simulink model "Lin_cartmodel"  (R2019b)
settings: Solver=VariableStepAuto  StartTime=0.0  StopTime=10.0  RelTol=1e-3
values from neighbouring files (symbols this model uses):
  A = Ab    [mainfile_solution.m]
  B = Bb    [mainfile_solution.m]
  C = Cb    [mainfile_solution.m]
  controller_enabled = 1    [mainfile_solution.m]
  K = place(A,B,p)    [mainfile_solution.m]
  L = place(A',C',p)'    [mainfile_solution.m]
  use_state_estimates = 1    [mainfile_solution.m]
  x0 = x0b    [mainfile_solution.m]
  x_bar = xb_bar    [mainfile_solution.m]
settings Model: Creator=n9182250  LastModifiedBy=n9182250
settings DebuggingCC: ArithmeticOperatorsInVariantConditions=warning
settings SFSimCC: CustomCodeUndefinedFunction=UseInterfaceOnly

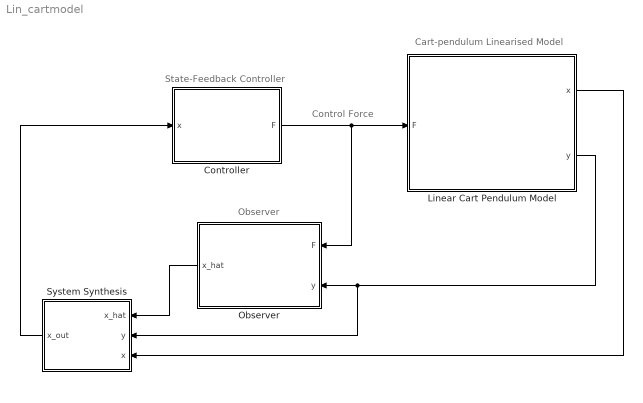
== system Lin_cartmodel ==
  note: Cart-pendulum Linearised Model
  note: Control Force
  note: State-Feedback Controller
  note: Observer
  Controller : Subsystem
  Linear Cart Pendulum Model : Subsystem
  Observer : Subsystem
  System Synthesis : Subsystem
  wires:
  Controller/1(F) -> Observer/1(F), Linear Cart Pendulum Model/1(F)
  Linear Cart Pendulum Model/2(y) -> System Synthesis/2(y), Observer/2(y)
  Observer/1(x_hat) -> System Synthesis/1(x_hat)
  Linear Cart Pendulum Model/1("x ") -> System Synthesis/3(x)
  System Synthesis/1(x_out) -> Controller/1(x)

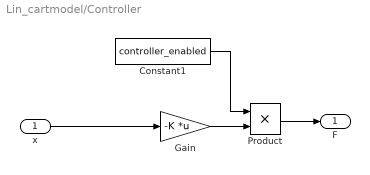
== system Lin_cartmodel/Controller ==
  x : Inport
  Constant1 : Constant  Value=controller_enabled
  Gain : Gain  Gain=-K  Multiplication=Matrix(K*u)
  Product : Product
  F : Outport
  wires:
  x/1 -> Gain/1
  Constant1/1 -> Product/1
  Gain/1 -> Product/2
  Product/1 -> F/1

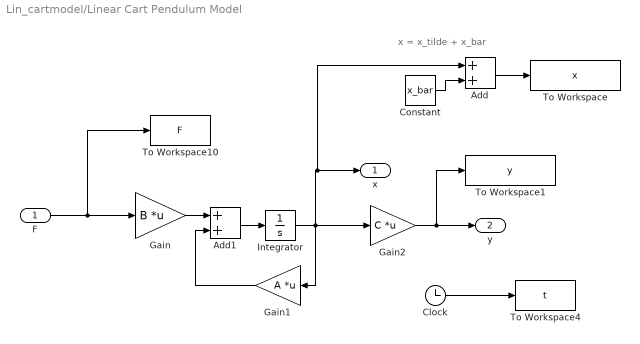
== system Lin_cartmodel/Linear Cart Pendulum Model ==
  note: x = x_tilde + x_bar
  F : Inport
  Add : Sum
  Add1 : Sum
  Clock : Clock
  Constant : Constant  Value=x_bar
  Gain : Gain  Gain=B  Multiplication=Matrix(K*u)
  Gain1 : Gain  Gain=A  Multiplication=Matrix(K*u)
  Gain2 : Gain  Gain=C  Multiplication=Matrix(K*u)
  Integrator : Integrator  InitialCondition=x0-x_bar
  To Workspace : ToWorkspace  VariableName=x  SampleTime=-1
  To Workspace1 : ToWorkspace  VariableName=y  SampleTime=-1
  To Workspace10 : ToWorkspace  VariableName=F  SampleTime=-1
  To Workspace4 : ToWorkspace  VariableName=t  SampleTime=-1
  "x " : Outport  VectorParamsAs1DForOutWhenUnconnected=off
  y : Outport  Port=2  VectorParamsAs1DForOutWhenUnconnected=off
  wires:
  F/1 -> To Workspace10/1, Gain/1
  Clock/1 -> To Workspace4/1
  Add/1 -> To Workspace/1
  Gain/1 -> Add1/1
  Gain1/1 -> Add1/2
  Add1/1 -> Integrator/1
  Integrator/1 -> Add/1, "x "/1, Gain2/1, Gain1/1
  Gain2/1 -> To Workspace1/1, y/1
  Constant/1 -> Add/2

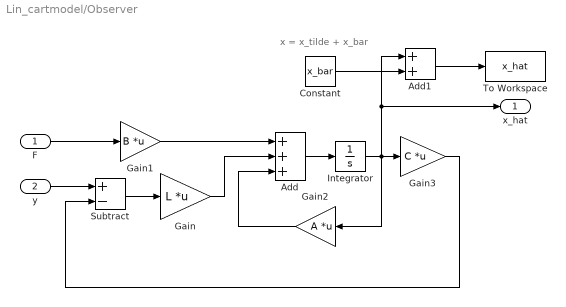
== system Lin_cartmodel/Observer ==
  note: x = x_tilde + x_bar
  F : Inport
  y : Inport  Port=2
  Add : Sum  Inputs=+++
  Add1 : Sum
  Constant : Constant  Value=x_bar
  Gain : Gain  Gain=L  Multiplication=Matrix(K*u)
  Gain1 : Gain  Gain=B  Multiplication=Matrix(K*u)
  Gain2 : Gain  Gain=A  Multiplication=Matrix(K*u)
  Gain3 : Gain  Gain=C  Multiplication=Matrix(K*u)
  Integrator : Integrator
  Subtract : Sum  Inputs=+-
  To Workspace : ToWorkspace  VariableName=x_hat  SampleTime=-1
  x_hat : Outport  VectorParamsAs1DForOutWhenUnconnected=off
  wires:
  y/1 -> Subtract/1
  Subtract/1 -> Gain/1
  F/1 -> Gain1/1
  Gain1/1 -> Add/1
  Gain/1 -> Add/2
  Add/1 -> Integrator/1
  Gain2/1 -> Add/3
  Gain3/1 -> Subtract/2
  Constant/1 -> Add1/2
  Integrator/1 -> Add1/1, x_hat/1, Gain2/1, Gain3/1
  Add1/1 -> To Workspace/1

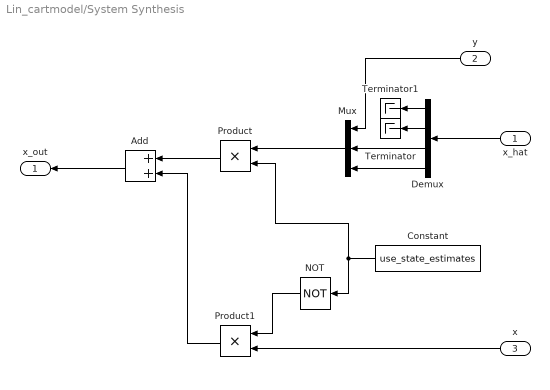
== system Lin_cartmodel/System Synthesis ==
  x_hat : Inport
  y : Inport  Port=2
  x : Inport  Port=3
  Add : Sum
  Constant : Constant  Value=use_state_estimates
  Demux : Demux
  Mux : Mux  Inputs=3
  NOT : Logic  Operator=NOT  IconShape=distinctive  AllPortsSameDT=off  OutDataTypeStr=boolean
  Product : Product
  Product1 : Product
  Terminator : Terminator
  Terminator1 : Terminator
  x_out : Outport
  wires:
  Demux/1 -> Terminator1/1
  Demux/2 -> Terminator/1
  Demux/3 -> Mux/2
  Demux/4 -> Mux/3
  y/1 -> Mux/1
  x_hat/1 -> Demux/1
  Mux/1 -> Product/1
  Constant/1 -> Product/2, NOT/1
  x/1 -> Product1/2
  NOT/1 -> Product1/1
  Add/1 -> x_out/1
  Product/1 -> Add/1
  Product1/1 -> Add/2
